simulink model "rc_node"  (Simulink 7.8)
settings: Solver=FixedStepDiscrete  SolverMode=SingleTasking  StartTime=0.0  StopTime=10.0  FixedStep=0.01  RelTol=1e-3
InitFcn:
  | clear all;
  | RcNodeInit
values from neighbouring files (symbols this model uses):
  MaxPwmIn = 0.0025    [RcNodeInit.m]
  T_step = 0.01    [RcNodeInit.m]
undefined symbols (not defined in the file or in its folder): Acs300SendThrottleCommand, ANmax, DataEEInitAndClear, DataStoreSaveParameters, DiscIntNeverNeededParam, Ecan1Init, IC1max, IC2max, IC7max, IC8max, Init_onlyOnce, Init_Reset, NodeTransmitStatus, RcNodeInit, RudderSendAngleCommand, RudderStartCalibration, TransmitStatus, u1, u2
libraries: simulink x35, dsPICdrivers x19, simulink_need_slupdate x1, ecan_dspic x1
(part 2 of 2)

== system rc_node/Manual Control/State outputs/If Action Subsystem5 ==
  Action Port : ActionPort  ActionType=else
  Constant1 : Constant  Value=false  OutDataTypeStr=Inherit: Inherit via back propagation
  LED1 : Outport  InitialOutput=false
  wires:
  Constant1/1 -> LED1/1

== system rc_node/Manual Control/State outputs/If Action Subsystem6 ==
  Pulse : Inport
  Action Port : ActionPort  ActionType=elseif
  LED1 : Outport  InitialOutput=false
  wires:
  Pulse/1 -> LED1/1

== system rc_node/Manual Control/Toggle manual control mode/RC transmitter is connected and the manual switch is engaged, so manual control is enabled. ==
  Action Port : ActionPort  ActionType=elseif
  Bitwise Operator : simulink/Logic and Bit Operations/Bitwise Operator  logicop=OR  UseBitMask=on  BitMask=1  BitMaskRealWorld=Stored Integer
  Data Store Read : DataStoreRead  DataStoreName=nodeStatus  SampleTime=T_step
  Data Store Write : DataStoreWrite  DataStoreName=nodeStatus
  wires:
  Data Store Read/1 -> Bitwise Operator/1
  Bitwise Operator/1 -> Data Store Write/1

== system rc_node/Manual Control/Toggle manual control mode/RC transmitter is connected, so update the status field ==
  Action Port : ActionPort  ActionType=elseif
  Bitwise Operator : simulink/Logic and Bit Operations/Bitwise Operator  logicop=OR  UseBitMask=on  BitMask=2  BitMaskRealWorld=Stored Integer
  Data Store Read : DataStoreRead  DataStoreName=nodeStatus  SampleTime=T_step
  Data Store Write : DataStoreWrite  DataStoreName=nodeStatus
  wires:
  Data Store Read/1 -> Bitwise Operator/1
  Bitwise Operator/1 -> Data Store Write/1

== system rc_node/Manual Control/Toggle manual control mode/RC transmitter is disconnected, so update the status field ==
  Action Port : ActionPort  ActionType=then
  Bitwise Operator1 : simulink/Logic and Bit Operations/Bitwise Operator  logicop=AND  UseBitMask=off  NumInputPorts=2  BitMask=~hex2dec('8')  BitMaskRealWorld=Stored Integer
  Bitwise Operator2 : simulink/Logic and Bit Operations/Bitwise Operator  logicop=NOT  UseBitMask=off  BitMask=~hex2dec('8')  BitMaskRealWorld=Stored Integer
  Constant : Constant  Value=2  OutDataTypeStr=Inherit: Inherit via back propagation
  Data Store Read1 : DataStoreRead  DataStoreName=nodeStatus  SampleTime=T_step
  Data Store Write1 : DataStoreWrite  DataStoreName=nodeStatus
  wires:
  Bitwise Operator1/1 -> Data Store Write1/1
  Data Store Read1/1 -> Bitwise Operator1/1
  Constant/1 -> Bitwise Operator2/1
  Bitwise Operator2/1 -> Bitwise Operator1/2

== system rc_node/Manual Control/Toggle manual control mode/RC transmitter is disconnected, therefore manual control is disabled. ==
  Action Port : ActionPort  ActionType=then
  Bitwise Operator1 : simulink/Logic and Bit Operations/Bitwise Operator  logicop=AND  UseBitMask=off  NumInputPorts=2  BitMask=~hex2dec('8')  BitMaskRealWorld=Stored Integer
  Bitwise Operator2 : simulink/Logic and Bit Operations/Bitwise Operator  logicop=NOT  UseBitMask=off  BitMask=~hex2dec('8')  BitMaskRealWorld=Stored Integer
  Constant : Constant  OutDataTypeStr=Inherit: Inherit via back propagation
  Data Store Read1 : DataStoreRead  DataStoreName=nodeStatus  SampleTime=T_step
  Data Store Write1 : DataStoreWrite  DataStoreName=nodeStatus
  wires:
  Bitwise Operator1/1 -> Data Store Write1/1
  Data Store Read1/1 -> Bitwise Operator1/1
  Constant/1 -> Bitwise Operator2/1
  Bitwise Operator2/1 -> Bitwise Operator1/2

== system rc_node/Manual Control/Radio Control Inputs/Calibrate/Calibration ==
  r : Inport
  t : Inport  Port=2
  Enable : EnablePort
  Data Store Read : DataStoreRead  DataStoreName=rcThrottleRange  SampleTime=T_step
  Data Store Read1 : DataStoreRead  DataStoreName=rcRudderRange  SampleTime=T_step
  Data Store Write : DataStoreWrite  DataStoreName=rcThrottleRange
  Data Store Write1 : DataStoreWrite  DataStoreName=rcRudderRange
  Update range from input : Subsystem
  Update range from input1 : Subsystem
  wires:
  Update range from input/1(newRange) -> Data Store Write1/1
  Data Store Read1/1 -> Update range from input/1(limitRange)
  r/1 -> Update range from input/2(newValue)
  Update range from input1/1(newRange) -> Data Store Write/1
  Data Store Read/1 -> Update range from input1/1(limitRange)
  t/1 -> Update range from input1/2(newValue)

== system rc_node/Manual Control/Radio Control Inputs/Calibrate/Detect calibration trigger ==
  note: This part checks for a mode change and checks that
      | it isn't the result of a disconnect. We don't want those
      | to accidently trigger a calibration.
  mode : Inport
  discon : Inport  Port=2
  Compare To Constant1 : simulink/Logic and Bit Operations/Compare To Constant  relop===  const=0  OutDataTypeStr=boolean
  Compute Calibration State : MATLAB Function  TreatAsAtomicUnit=on
  Data Store Memory : DataStoreMemory  DataStoreName=restoredCalibration  ReadBeforeWriteMsg=warning  WriteAfterWriteMsg=warning  WriteAfterReadMsg=warning  OutDataTypeStr=boolean
      settings: RTWStateStorageClass=ImportedExtern
  Data Store Read1 : DataStoreRead  DataStoreName=restoredCalibration  SampleTime=T_step
  Detect Change1 : simulink/Logic and Bit Operations/Detect Change  vinit=0  InputProcessing=Inherited  OutDataTypeStr=boolean
  IC : InitialCondition  Value=0
  Logical Operator : Logic  AllPortsSameDT=off  OutDataTypeStr=boolean
  calibrateState : Outport
  wires:
  mode/1 -> Detect Change1/1
  Logical Operator/1 -> Compute Calibration State/1(trigger)
  Detect Change1/1 -> Logical Operator/1
  Compare To Constant1/1 -> Logical Operator/2
  Compute Calibration State/1(state) -> IC/1
  Data Store Read1/1 -> Compute Calibration State/2(restoredCalibration)
  discon/1 -> Compare To Constant1/1
  IC/1 -> calibrateState/1

== system rc_node/Manual Control/Radio Control Inputs/Calibrate/Reset calibration range ==
  note: Reset the calibration range for each
      | channel before recalibration.
  Trigger : TriggerPort
  Constant1 : Constant  Value=[8000 8000]  OutDataTypeStr=Inherit: Inherit via back propagation  SampleTime=Inf
  Data Store Write : DataStoreWrite  DataStoreName=rcThrottleRange
  Data Store Write1 : DataStoreWrite  DataStoreName=rcRudderRange
  wires:
  Constant1/1 -> Data Store Write/1, Data Store Write1/1

== system rc_node/Manual Control/Radio Control Inputs/Calibrate/Save parameters ==
  Trigger : TriggerPort
  Save all parameters to memory [DataStore.c] : dsPICdrivers/OTHERS/C Function Call  Tag=dsPIC_dsPIC_CFunctionCall  FctUpdate=Output Function  fctName=DataStoreSaveParameters  INPUT_SIZE=1  INPUT1=--  INPUT2=--  INPUT3=--  OUTPUT_SIZE=1  OUTPUT1=--  SampleTime=-1  InputType=[ ]  OutputType=[ ]  FctDeclaration=extern void DataStoreSaveParameters();  FctCall=DataStoreSaveParameters();  OrderingInOutPopup=None  FctStart=None  FctStart_Name=Init_onlyOnce  FctStart_Declaration=inline extern void Init_onlyOnce();  FctStart_Call=Init_onlyOnce();  FctInit=None  FctInit_Name=Init_Reset  FctInit_Declaration=inline extern void Init_Reset();  FctInit_Call=Init_Reset();  PinDigitalInput=[]  PinDigitalOutput=[]  AnalogueInput=[]

== system rc_node/Manual Control/Radio Control Inputs/Subsystem/If Action Subsystem ==
  Action Port : ActionPort  ActionType=then
  Constant : Constant  Value=0  OutDataTypeStr=single
  Constant1 : Constant  Value=0  OutDataTypeStr=single
  Out1 : Outport  InitialOutput=50
  Out2 : Outport  Port=2  InitialOutput=50
  wires:
  Constant/1 -> Out1/1
  Constant1/1 -> Out2/1

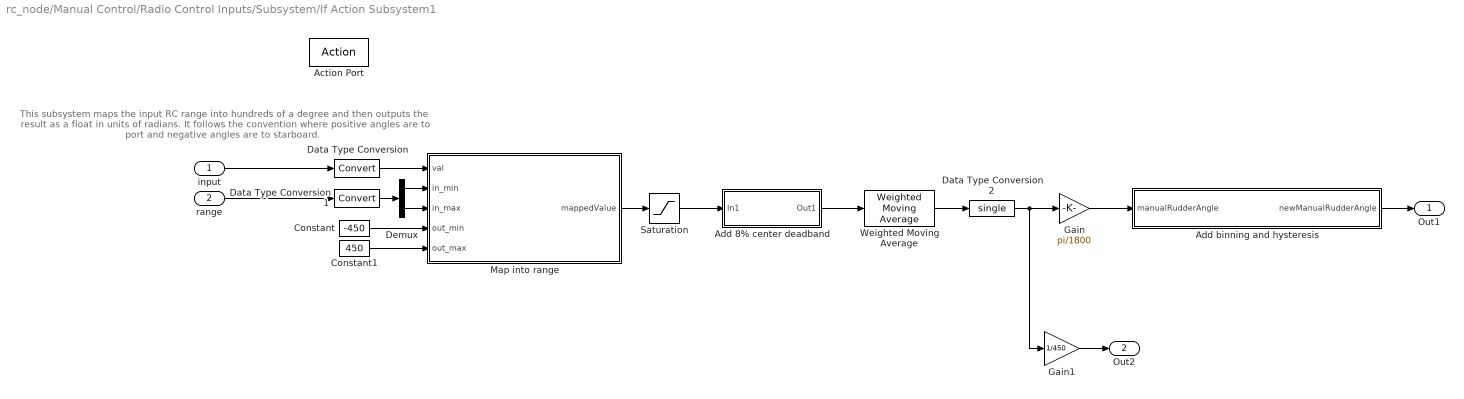
== system rc_node/Manual Control/Radio Control Inputs/Subsystem/If Action Subsystem1 ==
  note: This subsystem maps the input RC range into hundreds of a degree and then
      | outputs the result as a float in units of radians. It follows the convention where
      | positive angles are to port and negative angles are to starboard.
  input : Inport
  range : Inport  Port=2
  Action Port : ActionPort  ActionType=else
  Add 8% center deadband : Subsystem
  Add binning and hysteresis : MATLAB Function  TreatAsAtomicUnit=on
  Constant : Constant  Value=-450  OutDataTypeStr=Inherit: Inherit via back propagation
  Constant1 : Constant  Value=450  OutDataTypeStr=Inherit: Inherit via back propagation
  Data Type Conversion : DataTypeConversion
  Data Type Conversion1 : DataTypeConversion
  Data Type Conversion2 : DataTypeConversion  OutDataTypeStr=single  RndMeth=Simplest
  Demux : Demux  Outputs=2
  Gain : Gain  Gain=pi/1800
  Gain1 : Gain  Gain=1/450  OutDataTypeStr=single  RndMeth=Simplest
  Map into range : MATLAB Function  TreatAsAtomicUnit=on
  Saturation : Saturate  UpperLimit=450  LowerLimit=-450  OutDataTypeStr=int16  RndMeth=Simplest
  Weighted Moving Average : simulink_need_slupdate/Weighted Moving Average  mgainval=[.1 .1 .1 .1 .1 .1 .1 .1 .1 .1]  vinit=0.0  samptime=-1  OutDataTypeStr=Inherit: Inherit via back propagation  OutDataType=sfix(16)  OutScaling=2^-10  DoSatur=off  GainDataType=uint(16)  MatRadixGroup=Best Precision: Matrix-wise  GainScaling=2^-10
  Out1 : Outport  InitialOutput=50
  Out2 : Outport  Port=2  InitialOutput=50
  wires:
  Constant1/1 -> Map into range/5(out_max)
  Constant/1 -> Map into range/4(out_min)
  Demux/1 -> Map into range/2(in_min)
  Demux/2 -> Map into range/3(in_max)
  range/1 -> Data Type Conversion1/1
  Map into range/1(mappedValue) -> Saturation/1
  Data Type Conversion/1 -> Map into range/1(val)
  Data Type Conversion1/1 -> Demux/1
  input/1 -> Data Type Conversion/1
  Add 8% center deadband/1(Out1) -> Weighted Moving Average/1
  Saturation/1 -> Add 8% center deadband/1(In1)
  Gain/1 -> Add binning and hysteresis/1(manualRudderAngle)
  Data Type Conversion2/1 -> Gain/1, Gain1/1
  Weighted Moving Average/1 -> Data Type Conversion2/1
  Add binning and hysteresis/1(newManualRudderAngle) -> Out1/1
  Gain1/1 -> Out2/1

== system rc_node/Manual Control/Radio Control Inputs/Subsystem1/If Action Subsystem2 ==
  Action Port : ActionPort  ActionType=then
  Constant : Constant  Value=0  OutDataTypeStr=Inherit: Inherit via back propagation
  Constant1 : Constant  Value=0  OutDataTypeStr=single
  Out1 : Outport  InitialOutput=0
  Out2 : Outport  Port=2  InitialOutput=0
  wires:
  Constant/1 -> Out1/1
  Constant1/1 -> Out2/1

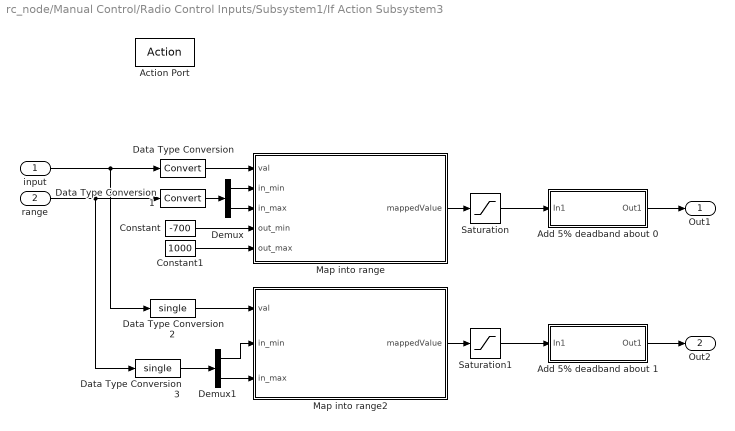
== system rc_node/Manual Control/Radio Control Inputs/Subsystem1/If Action Subsystem3 ==
  input : Inport
  range : Inport  Port=2
  Action Port : ActionPort  ActionType=else
  Add 5% deadband about 0 : Subsystem
  Add 5% deadband about 1 : Subsystem
  Constant : Constant  Value=-700  OutDataTypeStr=Inherit: Inherit via back propagation
  Constant1 : Constant  Value=1000  OutDataTypeStr=Inherit: Inherit via back propagation
  Data Type Conversion : DataTypeConversion
  Data Type Conversion1 : DataTypeConversion
  Data Type Conversion2 : DataTypeConversion  OutDataTypeStr=single
  Data Type Conversion3 : DataTypeConversion  OutDataTypeStr=single
  Demux : Demux  Outputs=2
  Demux1 : Demux  Outputs=2
  Map into range : MATLAB Function  TreatAsAtomicUnit=on
  Map into range2 : MATLAB Function  TreatAsAtomicUnit=on
  Saturation : Saturate  UpperLimit=1000  LowerLimit=-700  OutDataTypeStr=int16  RndMeth=Simplest
  Saturation1 : Saturate  UpperLimit=1.0  LowerLimit=-1.0  OutDataTypeStr=single  RndMeth=Simplest
  Out1 : Outport  InitialOutput=0
  Out2 : Outport  Port=2  InitialOutput=0
  wires:
  Constant1/1 -> Map into range/5(out_max)
  Constant/1 -> Map into range/4(out_min)
  Demux/1 -> Map into range/2(in_min)
  Demux/2 -> Map into range/3(in_max)
  range/1 -> Data Type Conversion1/1, Data Type Conversion3/1
  Map into range/1(mappedValue) -> Saturation/1
  Data Type Conversion/1 -> Map into range/1(val)
  Data Type Conversion1/1 -> Demux/1
  Saturation/1 -> Add 5% deadband about 0/1(In1)
  input/1 -> Data Type Conversion/1, Data Type Conversion2/1
  Add 5% deadband about 0/1(Out1) -> Out1/1
  Demux1/1 -> Map into range2/2(in_min)
  Demux1/2 -> Map into range2/3(in_max)
  Map into range2/1(mappedValue) -> Saturation1/1
  Saturation1/1 -> Add 5% deadband about 1/1(In1)
  Add 5% deadband about 1/1(Out1) -> Out2/1
  Data Type Conversion2/1 -> Map into range2/1(val)
  Data Type Conversion3/1 -> Demux1/1

== system rc_node/Manual Control/Radio Control Inputs/Trigger rudder calibration/ECAN1 TX ==
  Trigger : TriggerPort  PortDimensions=1
  Trigger rudder calibration [Rudder.c] : dsPICdrivers/OTHERS/C Function Call  Tag=dsPIC_dsPIC_CFunctionCall  FctUpdate=Output Function  fctName=RudderStartCalibration  INPUT_SIZE=1  INPUT1=--  INPUT2=--  INPUT3=--  OUTPUT_SIZE=1  OUTPUT1=--  SampleTime=-1  InputType=[ ]  OutputType=[ ]  FctDeclaration=extern void RudderStartCalibration();  FctCall=RudderStartCalibration();  OrderingInOutPopup=None  FctStart=None  FctStart_Name=Init_onlyOnce  FctStart_Declaration=inline extern void Init_onlyOnce();  FctStart_Call=Init_onlyOnce();  FctInit=None  FctInit_Name=Init_Reset  FctInit_Declaration=inline extern void Init_Reset();  FctInit_Call=Init_Reset();  PinDigitalInput=[]  PinDigitalOutput=[]  AnalogueInput=[]

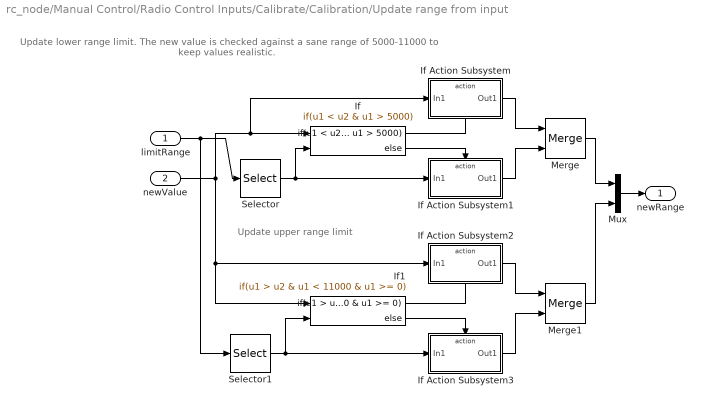
== system rc_node/Manual Control/Radio Control Inputs/Calibrate/Calibration/Update range from input ==
  note: Update lower range limit.
      | The new value is checked against a sane range of 5000-11000
      | to keep values realistic.
  note: Update upper range limit
  limitRange : Inport
  newValue : Inport  Port=2
  If : If  NumInputs=2  IfExpression=u1 < u2 & u1 > 5000
  If Action Subsystem : Subsystem  TreatAsAtomicUnit=on
  If Action Subsystem1 : Subsystem  TreatAsAtomicUnit=on
  If Action Subsystem2 : Subsystem  TreatAsAtomicUnit=on
  If Action Subsystem3 : Subsystem  TreatAsAtomicUnit=on
  If1 : If  NumInputs=2  IfExpression=u1 > u2 & u1 < 11000 & u1 >= 0
  Merge : Merge
  Merge1 : Merge
  Mux : Mux  Inputs=2
  Selector : Selector  InputPortWidth=2  IndexOptions=Index vector (dialog)  Indices=[1]  OutputSizes=1
  Selector1 : Selector  InputPortWidth=2  IndexOptions=Index vector (dialog)  Indices=[2]  OutputSizes=1
  newRange : Outport
  wires:
  Selector/1 -> If/2, If Action Subsystem1/1(In1)
  Selector1/1 -> If Action Subsystem3/1(In1), If1/2
  Mux/1 -> newRange/1
  Merge1/1 -> Mux/2
  Merge/1 -> Mux/1
  If Action Subsystem3/1(Out1) -> Merge1/2
  If Action Subsystem2/1(Out1) -> Merge1/1
  If1/2 -> If Action Subsystem3/Action
  If1/1 -> If Action Subsystem2/Action
  If Action Subsystem1/1(Out1) -> Merge/2
  If Action Subsystem/1(Out1) -> Merge/1
  If/2 -> If Action Subsystem1/Action
  If/1 -> If Action Subsystem/Action
  newValue/1 -> If Action Subsystem/1(In1), If/1, If Action Subsystem2/1(In1), If1/1
  limitRange/1 -> Selector/1, Selector1/1

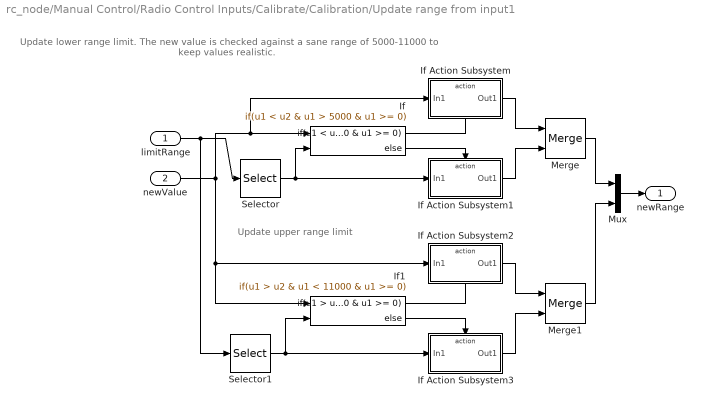
== system rc_node/Manual Control/Radio Control Inputs/Calibrate/Calibration/Update range from input1 ==
  note: Update lower range limit.
      | The new value is checked against a sane range of 5000-11000
      | to keep values realistic.
  note: Update upper range limit
  limitRange : Inport
  newValue : Inport  Port=2
  If : If  NumInputs=2  IfExpression=u1 < u2 & u1 > 5000 & u1 >= 0
  If Action Subsystem : Subsystem  TreatAsAtomicUnit=on
  If Action Subsystem1 : Subsystem  TreatAsAtomicUnit=on
  If Action Subsystem2 : Subsystem  TreatAsAtomicUnit=on
  If Action Subsystem3 : Subsystem  TreatAsAtomicUnit=on
  If1 : If  NumInputs=2  IfExpression=u1 > u2 & u1 < 11000 & u1 >= 0
  Merge : Merge
  Merge1 : Merge
  Mux : Mux  Inputs=2
  Selector : Selector  InputPortWidth=2  IndexOptions=Index vector (dialog)  Indices=[1]  OutputSizes=1
  Selector1 : Selector  InputPortWidth=2  IndexOptions=Index vector (dialog)  Indices=[2]  OutputSizes=1
  newRange : Outport
  wires:
  Selector/1 -> If/2, If Action Subsystem1/1(In1)
  Selector1/1 -> If Action Subsystem3/1(In1), If1/2
  Mux/1 -> newRange/1
  Merge1/1 -> Mux/2
  Merge/1 -> Mux/1
  If Action Subsystem3/1(Out1) -> Merge1/2
  If Action Subsystem2/1(Out1) -> Merge1/1
  If1/2 -> If Action Subsystem3/Action
  If1/1 -> If Action Subsystem2/Action
  If Action Subsystem1/1(Out1) -> Merge/2
  If Action Subsystem/1(Out1) -> Merge/1
  If/2 -> If Action Subsystem1/Action
  If/1 -> If Action Subsystem/Action
  newValue/1 -> If Action Subsystem/1(In1), If/1, If Action Subsystem2/1(In1), If1/1
  limitRange/1 -> Selector/1, Selector1/1

== system rc_node/Manual Control/Radio Control Inputs/Subsystem/If Action Subsystem1/Add 8% center deadband ==
  In1 : Inport
  If : If  IfExpression=u1 > -36 & u1 < 36
  If Action Subsystem : Subsystem  TreatAsAtomicUnit=on
  If Action Subsystem1 : Subsystem  TreatAsAtomicUnit=on
  Merge : Merge
  Out1 : Outport
  wires:
  In1/1 -> If Action Subsystem/1(In1), If/1
  If/2 -> If Action Subsystem/Action
  If/1 -> If Action Subsystem1/Action
  If Action Subsystem/1(Out1) -> Merge/2
  If Action Subsystem1/1(Out1) -> Merge/1
  Merge/1 -> Out1/1

== system rc_node/Manual Control/Radio Control Inputs/Subsystem1/If Action Subsystem3/Add 5% deadband about 0 ==
  In1 : Inport
  If : If  IfExpression=u1 < 43 & u1 > -43
  If Action Subsystem : Subsystem  TreatAsAtomicUnit=on
  If Action Subsystem1 : Subsystem  TreatAsAtomicUnit=on
  Merge : Merge
  Out1 : Outport
  wires:
  In1/1 -> If Action Subsystem/1(In1), If/1
  If/2 -> If Action Subsystem/Action
  If/1 -> If Action Subsystem1/Action
  If Action Subsystem1/1(Out1) -> Merge/1
  Merge/1 -> Out1/1
  If Action Subsystem/1(Out1) -> Merge/2

== system rc_node/Manual Control/Radio Control Inputs/Subsystem1/If Action Subsystem3/Add 5% deadband about 1 ==
  In1 : Inport
  If : If  IfExpression=u1 < single(0.025) & u1 > single(-0.025)
  If Action Subsystem : Subsystem  TreatAsAtomicUnit=on
  If Action Subsystem1 : Subsystem  TreatAsAtomicUnit=on
  Merge : Merge
  Out1 : Outport
  wires:
  If Action Subsystem/1(Out1) -> Merge/2
  Merge/1 -> Out1/1
  If Action Subsystem1/1(Out1) -> Merge/1
  If/1 -> If Action Subsystem1/Action
  If/2 -> If Action Subsystem/Action
  In1/1 -> If/1, If Action Subsystem/1(In1)

== system rc_node/Manual Control/Radio Control Inputs/Calibrate/Calibration/Update range from input/If Action Subsystem ==
  In1 : Inport
  Action Port : ActionPort  ActionType=then
  Out1 : Outport
  wires:
  In1/1 -> Out1/1

== system rc_node/Manual Control/Radio Control Inputs/Calibrate/Calibration/Update range from input/If Action Subsystem1 ==
  In1 : Inport
  Action Port : ActionPort  ActionType=else
  Out1 : Outport
  wires:
  In1/1 -> Out1/1

== system rc_node/Manual Control/Radio Control Inputs/Calibrate/Calibration/Update range from input/If Action Subsystem2 ==
  In1 : Inport
  Action Port : ActionPort  ActionType=then
  Out1 : Outport
  wires:
  In1/1 -> Out1/1

== system rc_node/Manual Control/Radio Control Inputs/Calibrate/Calibration/Update range from input/If Action Subsystem3 ==
  In1 : Inport
  Action Port : ActionPort  ActionType=else
  Out1 : Outport
  wires:
  In1/1 -> Out1/1

== system rc_node/Manual Control/Radio Control Inputs/Calibrate/Calibration/Update range from input1/If Action Subsystem ==
  In1 : Inport
  Action Port : ActionPort  ActionType=then
  Out1 : Outport
  wires:
  In1/1 -> Out1/1

== system rc_node/Manual Control/Radio Control Inputs/Calibrate/Calibration/Update range from input1/If Action Subsystem1 ==
  In1 : Inport
  Action Port : ActionPort  ActionType=else
  Out1 : Outport
  wires:
  In1/1 -> Out1/1

== system rc_node/Manual Control/Radio Control Inputs/Calibrate/Calibration/Update range from input1/If Action Subsystem2 ==
  In1 : Inport
  Action Port : ActionPort  ActionType=then
  Out1 : Outport
  wires:
  In1/1 -> Out1/1

== system rc_node/Manual Control/Radio Control Inputs/Calibrate/Calibration/Update range from input1/If Action Subsystem3 ==
  In1 : Inport
  Action Port : ActionPort  ActionType=else
  Out1 : Outport
  wires:
  In1/1 -> Out1/1

== system rc_node/Manual Control/Radio Control Inputs/Subsystem/If Action Subsystem1/Add 8% center deadband/If Action Subsystem ==
  In1 : Inport
  Action Port : ActionPort  ActionType=else
  Out1 : Outport
  wires:
  In1/1 -> Out1/1

== system rc_node/Manual Control/Radio Control Inputs/Subsystem/If Action Subsystem1/Add 8% center deadband/If Action Subsystem1 ==
  Action Port : ActionPort  ActionType=then
  Constant : Constant  Value=0  OutDataTypeStr=Inherit: Inherit via back propagation
  Out1 : Outport  InitialOutput=50
  wires:
  Constant/1 -> Out1/1

== system rc_node/Manual Control/Radio Control Inputs/Subsystem1/If Action Subsystem3/Add 5% deadband about 0/If Action Subsystem ==
  In1 : Inport
  Action Port : ActionPort  ActionType=else
  Out1 : Outport
  wires:
  In1/1 -> Out1/1

== system rc_node/Manual Control/Radio Control Inputs/Subsystem1/If Action Subsystem3/Add 5% deadband about 0/If Action Subsystem1 ==
  Action Port : ActionPort  ActionType=then
  Constant : Constant  Value=0  OutDataTypeStr=Inherit: Inherit via back propagation
  Out1 : Outport  InitialOutput=0
  wires:
  Constant/1 -> Out1/1

== system rc_node/Manual Control/Radio Control Inputs/Subsystem1/If Action Subsystem3/Add 5% deadband about 1/If Action Subsystem ==
  In1 : Inport
  Action Port : ActionPort  ActionType=else
  Out1 : Outport
  wires:
  In1/1 -> Out1/1

== system rc_node/Manual Control/Radio Control Inputs/Subsystem1/If Action Subsystem3/Add 5% deadband about 1/If Action Subsystem1 ==
  Action Port : ActionPort  ActionType=then
  Constant : Constant  Value=0  OutDataTypeStr=single
  Out1 : Outport  InitialOutput=0
  wires:
  Constant/1 -> Out1/1

== matlab function Manual Control/Radio Control Inputs/Trigger rudder calibration/Compute Calibration State ==
  data: trigger input boolean; out output double; mode input double; calState input double
function out = fcn(trigger, mode, calState)
%#codegen
% Trigger is the event trigger (a boolean) that needs to be toggled thrice
% to enter calibration mode.
% Mode needs to be high for the trigger to matter. It also needs to be
% turned off before calibration can be attempted again.

persistent countdownTimer transitionCounter internalState;

% Initialize persistent variables
if isempty(countdownTimer)
    countdownTimer = uint8(0);
    transitionCounter = uint8(0);
    internalState = uint8(0);
end

out = false;

% Do the state processing:
switch internalState
    case 0 % Off
        % When we get a trigger, if we're in the correct mode, go into state 1 clearing the timer for use
        % We also check if the calibration state is either calibrated or
        % in the post-calibration transition mode. This prevents rudder
        % calibration when the RC transmitter isn't calibrated.
        if trigger && mode && calState > 2
            transitionCounter = uint8(1);
            internalState = uint8(1);
            countdownTimer = uint8(0);
        end
    case 1 % Transition mode
        % Here we just keep a timer going and once it expires we go back to off,
        % otherwise we count transitions until we've hit 3 then we go to calibration mode.
        countdownTimer = countdownTimer + 1;
        if ~mode
            internalState = uint8(0);
        elseif countdownTimer > 150
            internalState = uint8(0);
        elseif trigger
            transitionCounter = transitionCounter + 1;
        
            % Once we've hit three transitions, trigger the calibration!
            if transitionCounter == uint8(3)
                internalState = uint8(2);
                out = true;
            end
        end
    case 2 % Calibrated
        % Here we just sit and do nothing. We don't allow recalibration
        % until the mode is disabled. Once the mode is disabled, we go back
        % to the first state so that this recalibration can be triggered.
        if ~mode
            internalState = uint8(0);
        end
end

== matlab function Manual Control/Radio Control Inputs/Subsystem1/If Action Subsystem3/Map into range2 ==
  data: mappedValue output single; val input single; in_min input single; in_max input single
function mappedValue = map(val, in_min, in_max)
%#codegen
    mappedValue = (val - ((in_max + in_min) / 2)) / ((in_max - in_min) / 2);
end

== matlab function Manual Control/Radio Control Inputs/Calibrate/Detect calibration trigger/Compute Calibration State ==
  data: trigger input boolean; state output uint8; restoredCalibration input double
function state = fcn(trigger, restoredCalibration)
%#codegen

persistent countdownTimer transitionCounter internalState;

% Initialize persistent variables
if isempty(countdownTimer)
    countdownTimer = uint8(0);
    transitionCounter = uint8(0);
    
    if restoredCalibration
        internalState = uint8(3);
    else
        internalState = uint8(0);
    end
end

% Do the state processing:
switch internalState
    case 0 % Off
        % When we get a trigger, go into state 1 clearing the timer for use
        if trigger
            transitionCounter = uint8(1);
            internalState = uint8(1);
            countdownTimer = uint8(0);
        end
    case 1 % Transition mode
        % Here we just keep a timer going and once it expires we go back to off,
        % otherwise we count transitions until we've hit 3 then we go to calibration mode.
        countdownTimer = countdownTimer + 1;
        if countdownTimer > 150
            internalState = uint8(0);
        elseif trigger
            transitionCounter = transitionCounter + 1;
        
            % Once we've hit three transitions, we're in calibration mode!
            if transitionCounter == uint8(3)
                internalState = uint8(2);
            end
        end
    case 2 % Calibration mode
        % On the trigger, go into a calibrated mode.
        if trigger
            internalState = uint8(3);
        end
    case 3 % Calibrated
        % When we get a trigger, go into state 4 clearing the timer for use
        if trigger
            transitionCounter = uint8(1);
            internalState = uint8(4);
            countdownTimer = uint8(0);
        end
    case 4 % Transition mode (post-calibration)
        % Here we just keep a timer going and once it expires we go back to calibrated,
        % otherwise we count transitions until we've hit 3 then we go to calibration mode.
        countdownTimer = countdownTimer + 1;
        if countdownTimer > 150
            internalState = uint8(3);
        elseif trigger
            transitionCounter = transitionCounter + 1;
        
            % Once we've hit three transitions, we're in calibration mode!
            if transitionCounter == uint8(3)
                internalState = uint8(2);
            end
        end
end

% Output the internal state
state = internalState;

== matlab function Manual Control/Radio Control Inputs/Subsystem/If Action Subsystem1/Map into range ==
  data: mappedValue output int32; val input int32; in_min input int32; in_max input int32; out_min input int32; out_max input int32
function mappedValue = map(val, in_min, in_max, out_min, out_max)
%#codegen
% Pulled from: http://www.arduino.cc/cgi-bin/yabb2/YaBB.pl?num=1289758376, first post
% This is a basic integer implementation of a map() function.
% NOTE: There can be integer overflow in the first multiplication.

  mappedValue = (val - in_min) * (out_max - out_min) / (in_max - in_min) + out_min;

end

== matlab function Manual Control/Radio Control Inputs/Subsystem1/If Action Subsystem3/Map into range ==
  data: mappedValue output int32; val input int32; in_min input int32; in_max input int32; out_min input int32; out_max input int32
function mappedValue = map(val, in_min, in_max, out_min, out_max)
%#codegen
% Pulled from: http://www.arduino.cc/cgi-bin/yabb2/YaBB.pl?num=1289758376, first post
% This is a basic integer implementation of a map() function.
% NOTE: There can be integer overflow in the first multiplication.

  mappedValue = (val - in_min) * (out_max - out_min) / (in_max - in_min) + out_min;

end

== matlab function Manual Control/Radio Control Inputs/Subsystem/If Action Subsystem1/Add binning and hysteresis ==
  data: manualRudderAngle input double; newManualRudderAngle output double
function newManualRudderAngle = fcn(manualRudderAngle)
%#codegen
% This function takes in a value from -.7854 to .7854 and adds binning and hysteresis
% to it. The goal is to stabilize the input and make it easier to control.
% The bins are roughly as follows (negative values are a mirror image):
% (0),  (6),  (12),  (18),  (23),  (28),  (33),  (39),  (45)
% 0-5.9, 6-10.9, 11-15.9, 16-20.9, 21-25.9, 26-30.9, 31-35.9, 36-40.9, 41-45

% Hysteresis follows an offset of 2.5 degrees. So to transition from the 0 
% degree bin to the 6 degree bin, the input must have reached 8.5 degrees.
% To transition back it needs to hit 2.5 degrees.

% This code only moves a single bin per timestep. This shouldn't be a 
% problem considering how quick the timesteps are (100Hz) that I don't think
% that the user will ever notice it.

% Store the start of each bin range in radians.
transitions = single([0 6 11 16 21 26 31 36 40]*pi/180);

% Store the mapped rudder angles for each bin
binAngles = single([0 6 12 18 23 28 33 39 45]*pi/180);

% Keep track of some properties from the input. Segregating it like this
% makes the code cleaner.
tempRudderAngle = single(abs(manualRudderAngle));

% Keep track of which bin we're in so that hysteresis can be done. This is
% NOT a stateless algorithm. We initialize into the 0 bin.
persistent bin;

if isempty(bin)
    bin = uint8(1);
end

% Make sure the next higher bin exists and then check if we should move into
% it. This code only moves one bin per timestep.
if bin + uint8(1) <= length(transitions)
    if tempRudderAngle > transitions(bin + 1) + single(0.0349)
        bin = bin + uint8(1);
    end
end

% Make sure the next lower bin exists and then check if we should move into
% it. This code only moves one bin per timestep.
if bin - uint8(1) > 0
    if tempRudderAngle < transitions(bin) - single(0.0436)
        bin = bin - uint8(1);
    end
end

% Finally here we output the mapped value. We account for whether the output
% should be negative based on whether the input was.
if manualRudderAngle < 0
    newManualRudderAngle = -binAngles(bin);
else
    newManualRudderAngle = binAngles(bin);
end

== matlab function Manual Control/Radio Control Inputs/Clear to 0 if Disconnect/Set the throttle to 0 if it's only a heartbeat ==
  data: u input double; y output double
function y = fcn(u)
%#codegen

if u < uint16(4700)
    y = uint16(0);
else
    y = u;
end
